simulink model "UKF_10hz"  (Simulink 8.3)
settings: Solver=FixedStepDiscrete  StartTime=0.0  StopTime=run_time  FixedStep=.01  RelTol=1e-3
values from neighbouring files (symbols this model uses):
  B_bias = [0 0 0]    [Initialize_UKF_Function.m]
  B_Init_Inertial = wrldmagm(Alt, Lat, Long, 2013)*1E-9    [Initialize_UKF_Function.m]
  I_c = [3.4 3.4 1.9]    [Initialize_UKF_Function.m]    (also in UKF_quaternion_withBias.m)
  NED_Init = dcmecef2ned(Lat, Long)*ECEF_Init    [Initialize_UKF_Function.m]
  q_i_s0 = init_attitude    [Initialize_UKF_Function.m]
  q_s_c = [1 0 0 0]    [Initialize_UKF_Function.m]    (also in Satellite2Controller_Conversion.m = dcm2quat(R); UKF_quaternion_withBias.m = [1; 0; 0; 0])
  Time_Start = 0    [Initialize_UKF_Function.m]
  Torque_s = [0 0 0]    [Initialize_UKF_Function.m]
  Ts = .1    (= 0.1)    [Initialize_UKF_Function.m]
  w_bias = 0*[0.5 0.2 0.15]    [Initialize_UKF_Function.m]    (also in UKF_quaternion_withBias.m = zeros(3,1))
  w_init_s = [rand_w_x rand_w_y rand_w_z]    [Initialize_UKF_Function.m]
undefined symbols (not defined in the file or in its folder): aeroassertmsg, c, cd, dyear, Earth, epoch, fm, fn, k, maxdef, Newton, Raphson, sgp4, snorm, WGS84
libraries: commnoisgen2 x6, aerolibtransform2 x4, aerolibconvert2 x4, simulink x3, dspmtrx3 x1, aerolibgravitysys x1, aerolibutil x1
(part 2 of 3)

== system UKF_10hz/Orbital Enviroment/Orbital Model/Subsystem/World Magnetic Model 2010/geomag/Rotate magnetic vector components  to geodetic from spherical and  compute declination, inclination  and total intensity/Compute declination, inclination,  and total intensity ==
  by : Inport
  bx : Inport  Port=2
  bz : Inport  Port=3
  Angle Conversion1 : aerolibconvert2/Angle Conversion  IU=rad  OU=deg
  Angle Conversion2 : aerolibconvert2/Angle Conversion  IU=rad  OU=deg
  Product : Product  SaturateOnIntegerOverflow=on  OutDataTypeStr=Inherit: Same as first input
  Product1 : Product  SaturateOnIntegerOverflow=on  OutDataTypeStr=Inherit: Same as first input
  Product2 : Product  SaturateOnIntegerOverflow=on  OutDataTypeStr=Inherit: Same as first input
  Sum : Sum  Inputs=|++  SaturateOnIntegerOverflow=on
  Sum1 : Sum  Inputs=++|  SaturateOnIntegerOverflow=on
  Trigonometric Function : Trigonometry  Operator=atan2
  Trigonometric Function1 : Trigonometry  Operator=atan2
  sqrt : Sqrt  AlgorithmType=Newton-Raphson  SaturateOnIntegerOverflow=on
  sqrt1 : Sqrt  AlgorithmType=Newton-Raphson  SaturateOnIntegerOverflow=on
  dec : Outport
  dip : Outport  Port=2
  ti : Outport  Port=3
  wires:
  sqrt/1 -> ti/1
  by/1 -> Product/1, Product/2, Trigonometric Function1/1
  bx/1 -> Product1/1, Product1/2, Trigonometric Function1/2
  bz/1 -> Product2/1, Product2/2, Trigonometric Function/1
  Product/1 -> Sum/1
  Product1/1 -> Sum/2
  Sum/1 -> Sum1/2, sqrt1/1
  Product2/1 -> Sum1/1
  Sum1/1 -> sqrt/1
  sqrt1/1 -> Trigonometric Function/2
  Trigonometric Function/1 -> Angle Conversion2/1
  Angle Conversion2/1 -> dip/1
  Trigonometric Function1/1 -> Angle Conversion1/1
  Angle Conversion1/1 -> dec/1

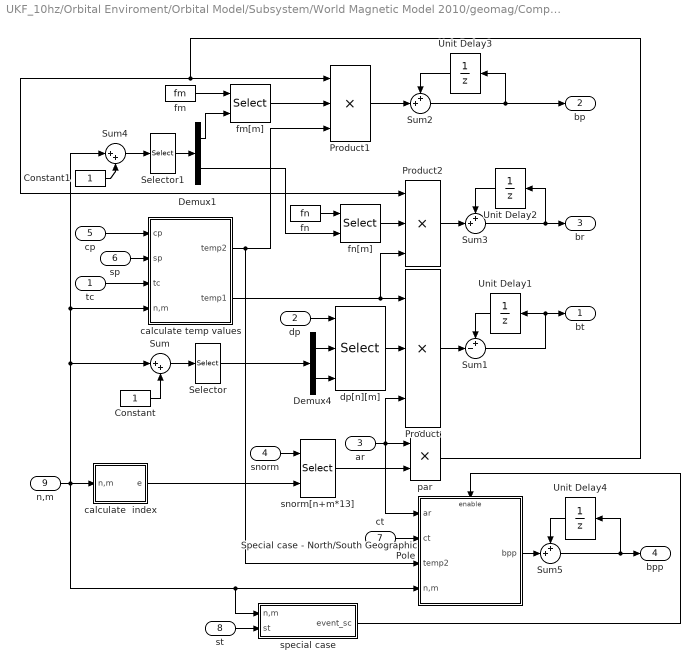
== system UKF_10hz/Orbital Enviroment/Orbital Model/Subsystem/World Magnetic Model 2010/geomag/Compute magnetic vector in spherical coordinates/For Iterator Subsystem/Accumulate terms of the  spherical harmonic expansion ==
  tc : Inport
  dp : Inport  Port=2
  ar : Inport  Port=3
  snorm : Inport  Port=4
  cp : Inport  Port=5
  sp : Inport  Port=6
  ct : Inport  Port=7
  st : Inport  Port=8
  n,m : Inport  Port=9
  Constant : Constant  OutDataTypeStr=Inherit: Inherit via back propagation
  Constant1 : Constant  OutDataTypeStr=Inherit: Inherit via back propagation
  Demux1 : Demux  Outputs=2
  Demux4 : Demux  Outputs=2
  Product : Product  Inputs=3  SaturateOnIntegerOverflow=on  OutDataTypeStr=Inherit: Same as first input
  Product1 : Product  Inputs=3  SaturateOnIntegerOverflow=on  OutDataTypeStr=Inherit: Same as first input
  Product2 : Product  Inputs=3  SaturateOnIntegerOverflow=on  OutDataTypeStr=Inherit: Same as first input
  Selector : Selector  InputPortWidth=2  Indices=[2 1]
  Selector1 : Selector  InputPortWidth=2  Indices=[2 1]
  Special case - North/South Geographic Pole : Subsystem  TreatAsAtomicUnit=on
  Sum : Sum  Inputs=|++  SaturateOnIntegerOverflow=on
  Sum1 : Sum  Inputs=+-|  SaturateOnIntegerOverflow=on
  Sum2 : Sum  Inputs=++|  SaturateOnIntegerOverflow=on
  Sum3 : Sum  Inputs=++|  SaturateOnIntegerOverflow=on
  Sum4 : Sum  Inputs=|++  SaturateOnIntegerOverflow=on
  Sum5 : Sum  Inputs=++|  SaturateOnIntegerOverflow=on
  Unit Delay{1..4} (4 alike) : UnitDelay  SampleTime=-1
  calculate  index : Subsystem
  calculate temp values : Subsystem
  dp[n][m] : Selector  NumberOfDimensions=2  InputPortWidth=maxdef+1  IndexOptions=Index vector (port),Index vector (port)  Indices=1,1
  fm : Constant  Value=fm  OutDataTypeStr=Inherit: Inherit via back propagation
  fm[m] : Selector  InputPortWidth=maxdef+1  IndexOptions=Index vector (port)  Indices=[1 3]
  fn : Constant  Value=fn  OutDataTypeStr=Inherit: Inherit via back propagation
  fn[m] : Selector  InputPortWidth=maxdef+1  IndexOptions=Index vector (port)  Indices=[1 3]
  par : Product  SaturateOnIntegerOverflow=on  OutDataTypeStr=Inherit: Same as first input
  snorm[n+m*13] : Selector  InputPortWidth=(maxdef+1)*(maxdef+1)  IndexOptions=Index vector (port)  Indices=[1 3]
  special case : Subsystem
  bt : Outport
  bp : Outport  Port=2
  br : Outport  Port=3
  bpp : Outport  Port=4
  wires:
  Special case - North/South Geographic Pole/1(bpp) -> Sum5/2
  Sum5/1 -> bpp/1, Unit Delay4/1
  Unit Delay4/1 -> Sum5/1
  snorm[n+m*13]/1 -> par/2
  ar/1 -> Product/3, par/1, Special case - North/South Geographic Pole/1(ar)
  calculate  index/1(e) -> snorm[n+m*13]/2
  calculate temp values/2(temp1) -> Product2/3, Product/1
  dp[n][m]/1 -> Product/2
  Product/1 -> Sum1/2
  Sum1/1 -> bt/1, Unit Delay1/1
  Unit Delay1/1 -> Sum1/1
  calculate temp values/1(temp2) -> Product1/3, Special case - North/South Geographic Pole/3(temp2)
  par/1 -> Product2/1, Product1/1
  fn/1 -> fn[m]/1
  fm/1 -> fm[m]/1
  Product1/1 -> Sum2/2
  Sum2/1 -> bp/1, Unit Delay3/1
  Unit Delay3/1 -> Sum2/1
  dp/1 -> dp[n][m]/1
  snorm/1 -> snorm[n+m*13]/1
  n,m/1 -> calculate  index/1(n,m), Sum/1, calculate temp values/4(n,m), Sum4/1, Special case - North/South Geographic Pole/4(n,m), special case/1(n,m)
  cp/1 -> calculate temp values/1(cp)
  sp/1 -> calculate temp values/2(sp)
  fn[m]/1 -> Product2/2
  fm[m]/1 -> Product1/2
  Product2/1 -> Sum3/2
  Sum3/1 -> br/1, Unit Delay2/1
  Unit Delay2/1 -> Sum3/1
  tc/1 -> calculate temp values/3(tc)
  Sum/1 -> Selector/1
  Constant/1 -> Sum/2
  Selector/1 -> Demux4/1
  Demux4/1 -> dp[n][m]/2
  Demux4/2 -> dp[n][m]/3
  Constant1/1 -> Sum4/2
  Sum4/1 -> Selector1/1
  Selector1/1 -> Demux1/1
  Demux1/1 -> fm[m]/2
  Demux1/2 -> fn[m]/2
  ct/1 -> Special case - North/South Geographic Pole/2(ct)
  st/1 -> special case/2(st)
  special case/1(event_sc) -> Special case - North/South Geographic Pole/Enable

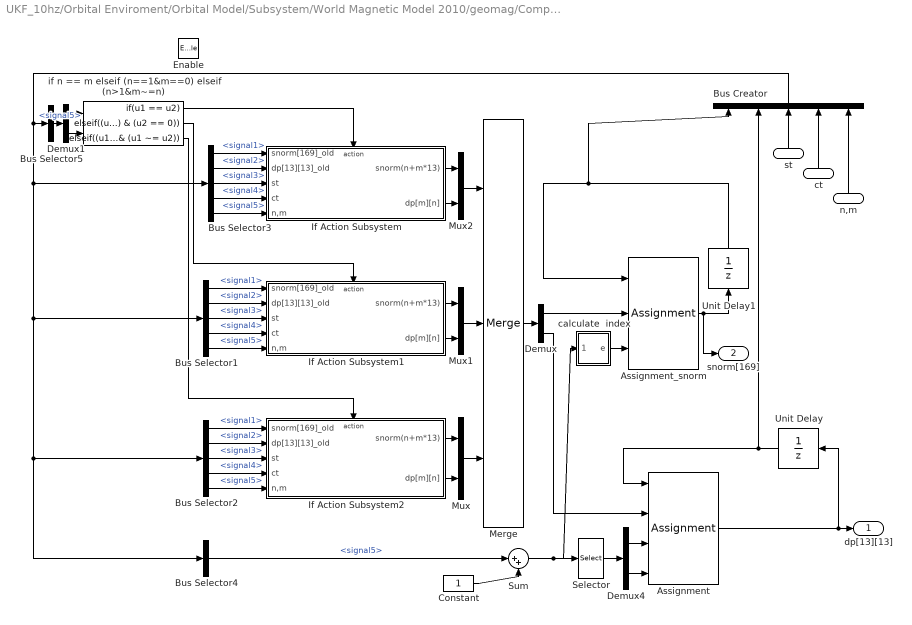
== system UKF_10hz/Orbital Enviroment/Orbital Model/Subsystem/World Magnetic Model 2010/geomag/Compute magnetic vector in spherical coordinates/For Iterator Subsystem/Compute unnormalized associated  legendre polynomials and  derivatives via recursion relations ==
  n,m : Inport
  st : Inport  Port=2
  ct : Inport  Port=3
  Enable : EnablePort  PropagateVarSize=During execution
  Assignment : Assignment  NumberOfDimensions=2  DiagnosticForDimensions=Error  IndexOptions=Index vector (port),Index vector (port)  Indices=1,1  OutputSizes=1,1
  Assignment_snorm : Assignment  DiagnosticForDimensions=Error  IndexOptions=Index vector (port)  OutputSizes=[1 1]
  Bus Creator : BusCreator  Inputs=5
  Bus Selector1 : BusSelector  OutputSignals=signal1,signal2,signal3,signal4,signal5
  Bus Selector2 : BusSelector  OutputSignals=signal1,signal2,signal3,signal4,signal5
  Bus Selector3 : BusSelector  OutputSignals=signal1,signal2,signal3,signal4,signal5
  Bus Selector4 : BusSelector  OutputSignals=signal5
  Bus Selector5 : BusSelector  OutputSignals=signal5
  Constant : Constant  OutDataTypeStr=Inherit: Inherit via back propagation
  Demux : Demux  Outputs=2
  Demux1 : Demux  Outputs=2
  Demux4 : Demux  Outputs=2
  If Action Subsystem : Subsystem  TreatAsAtomicUnit=on
  If Action Subsystem1 : Subsystem  TreatAsAtomicUnit=on
  If Action Subsystem2 : Subsystem  TreatAsAtomicUnit=on
  Merge : Merge  Inputs=3
  Mux : Mux  Inputs=2
  Mux1 : Mux  Inputs=2
  Mux2 : Mux  Inputs=2
  Selector : Selector  InputPortWidth=2  Indices=[2 1]
  Sum : Sum  Inputs=|++  SaturateOnIntegerOverflow=on
  Unit Delay : UnitDelay  InitialCondition=zeros(maxdef+1,maxdef+1)  SampleTime=-1
  Unit Delay1 : UnitDelay  InitialCondition=snorm  SampleTime=-1
  calculate  index : Subsystem
  if n == m elseif (n==1&m==0) elseif (n>1&m~=n) : If  NumInputs=2  IfExpression=u1 == u2  ElseIfExpressions=(u1 == 1) & (u2 == 0),(u1 >1) & (u1 ~= u2)  ShowElse=off
  dp[13][13] : Outport
  snorm[169] : Outport  Port=2
  wires:
  Constant/1 -> Sum/2
  if n == m elseif (n==1&m==0) elseif (n>1&m~=n)/1 -> If Action Subsystem/Action
  Assignment/1 -> dp[13][13]/1, Unit Delay/1
  if n == m elseif (n==1&m==0) elseif (n>1&m~=n)/2 -> If Action Subsystem1/Action
  if n == m elseif (n==1&m==0) elseif (n>1&m~=n)/3 -> If Action Subsystem2/Action
  Assignment_snorm/1 -> Unit Delay1/1, snorm[169]/1
  calculate  index/1(e) -> Assignment_snorm/3
  If Action Subsystem2/1(snorm(n+m*13)) -> Mux/1
  If Action Subsystem2/2(dp[m][n]) -> Mux/2
  If Action Subsystem1/1(snorm(n+m*13)) -> Mux1/1
  If Action Subsystem1/2(dp[m][n]) -> Mux1/2
  If Action Subsystem/1(snorm(n+m*13)) -> Mux2/1
  If Action Subsystem/2(dp[m][n]) -> Mux2/2
  Mux2/1 -> Merge/1
  Mux1/1 -> Merge/2
  Mux/1 -> Merge/3
  Merge/1 -> Demux/1
  Demux/2 -> Assignment/2
  Demux/1 -> Assignment_snorm/2
  Bus Selector2/1 -> If Action Subsystem2/1(snorm[169]_old)  "<signal1>"
  Bus Selector2/2 -> If Action Subsystem2/2(dp[13][13]_old)  "<signal2>"
  Bus Selector2/3 -> If Action Subsystem2/3(st)  "<signal3>"
  Bus Selector2/4 -> If Action Subsystem2/4(ct)  "<signal4>"
  Bus Selector1/1 -> If Action Subsystem1/1(snorm[169]_old)  "<signal1>"
  Bus Selector1/2 -> If Action Subsystem1/2(dp[13][13]_old)  "<signal2>"
  Bus Selector1/3 -> If Action Subsystem1/3(st)  "<signal3>"
  Bus Selector1/4 -> If Action Subsystem1/4(ct)  "<signal4>"
  Bus Selector3/1 -> If Action Subsystem/1(snorm[169]_old)  "<signal1>"
  Bus Selector3/2 -> If Action Subsystem/2(dp[13][13]_old)  "<signal2>"
  Bus Selector3/3 -> If Action Subsystem/3(st)  "<signal3>"
  Bus Selector3/4 -> If Action Subsystem/4(ct)  "<signal4>"
  st/1 -> Bus Creator/3
  ct/1 -> Bus Creator/4
  Bus Creator/1 -> Bus Selector1/1, Bus Selector2/1, Bus Selector4/1, Bus Selector3/1, Bus Selector5/1
  Sum/1 -> calculate  index/1(n,m), Selector/1
  Demux4/1 -> Assignment/3
  Demux4/2 -> Assignment/4
  Selector/1 -> Demux4/1
  n,m/1 -> Bus Creator/5
  Bus Selector1/5 -> If Action Subsystem1/5(n,m)  "<signal5>"
  Bus Selector2/5 -> If Action Subsystem2/5(n,m)  "<signal5>"
  Bus Selector3/5 -> If Action Subsystem/5(n,m)  "<signal5>"
  Bus Selector4/1 -> Sum/1  "<signal5>"
  Unit Delay/1 -> Assignment/1, Bus Creator/2
  Unit Delay1/1 -> Bus Creator/1, Assignment_snorm/1
  Demux1/1 -> if n == m elseif (n==1&m==0) elseif (n>1&m~=n)/1
  Demux1/2 -> if n == m elseif (n==1&m==0) elseif (n>1&m~=n)/2
  Bus Selector5/1 -> Demux1/1  "<signal5>"

== system UKF_10hz/Orbital Enviroment/Orbital Model/Subsystem/World Magnetic Model 2010/geomag/Compute magnetic vector in spherical coordinates/For Iterator Subsystem/Time adjust the gauss coefficients ==
  n : Inport
  m : Inport  Port=2
  dt : Inport  Port=3
  Enable : EnablePort  PropagateVarSize=During execution
  Assignment : Assignment  NumberOfDimensions=2  DiagnosticForDimensions=Error  IndexOptions=Index vector (port),Index vector (port)  Indices=1,1  OutputSizes=1,1
  Bus Creator : BusCreator  Inputs=5
  Bus Selector1 : BusSelector  OutputSignals=signal1,signal2,signal3,signal4,signal5
  If Action Subsystem : Subsystem  TreatAsAtomicUnit=on
  Sum2 : Sum  Inputs=|++  OutDataTypeStr=Inherit: Inherit via back propagation  SaturateOnIntegerOverflow=on
  Unit Delay : UnitDelay  InitialCondition=zeros(maxdef+1,maxdef+1)  SampleTime=-1
  c[maxdef][maxdef] : Constant  Value=c  OutDataTypeStr=Inherit: Inherit via back propagation
  cd[maxdef][maxdef] : Constant  Value=cd  OutDataTypeStr=Inherit: Inherit via back propagation
  if (m~=0) : Subsystem
  tc[13][13] : Outport
  wires:
  m/1 -> Bus Creator/1
  Bus Selector1/1 -> If Action Subsystem/1(m)  "<signal1>"
  Bus Selector1/2 -> If Action Subsystem/2(n)  "<signal2>"
  Bus Selector1/3 -> If Action Subsystem/3(dt)  "<signal3>"
  Bus Selector1/5 -> If Action Subsystem/5(cd)  "<signal5>"
  n/1 -> Bus Creator/2
  dt/1 -> Bus Creator/3
  c[maxdef][maxdef]/1 -> Bus Creator/4
  cd[maxdef][maxdef]/1 -> Bus Creator/5
  Assignment/1 -> Unit Delay/1, Sum2/1
  If Action Subsystem/1(tc) -> Assignment/2
  If Action Subsystem/2(row) -> Assignment/3
  If Action Subsystem/3(col) -> Assignment/4
  Bus Creator/1 -> if (m~=0)/1(bus), Bus Selector1/1
  Bus Selector1/4 -> If Action Subsystem/4(c)  "<signal4>"
  if (m~=0)/1(tc[13][13]) -> Sum2/2
  Unit Delay/1 -> Assignment/1
  Sum2/1 -> tc[13][13]/1

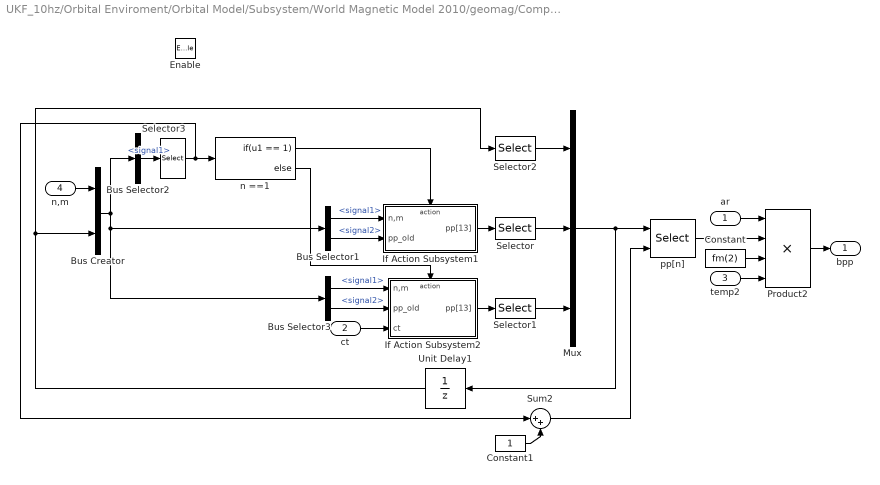
== system UKF_10hz/Orbital Enviroment/Orbital Model/Subsystem/World Magnetic Model 2010/geomag/Compute magnetic vector in spherical coordinates/For Iterator Subsystem/Accumulate terms of the  spherical harmonic expansion/Special case - North/South Geographic Pole ==
  ar : Inport
  ct : Inport  Port=2
  temp2 : Inport  Port=3
  n,m : Inport  Port=4
  Enable : EnablePort  PropagateVarSize=During execution
  Bus Creator : BusCreator  Inputs=2
  Bus Selector1 : BusSelector  OutputSignals=signal1,signal2
  Bus Selector2 : BusSelector  OutputSignals=signal1
  Bus Selector3 : BusSelector  OutputSignals=signal1,signal2
  Constant : Constant  Value=fm(2)  OutDataTypeStr=Inherit: Inherit via back propagation
  Constant1 : Constant
  If Action Subsystem1 : Subsystem
  If Action Subsystem2 : Subsystem
  Mux : Mux  Inputs=3
  Product2 : Product  Inputs=4  SaturateOnIntegerOverflow=on  OutDataTypeStr=Inherit: Same as first input
  Selector : Selector  InputPortWidth=maxdef+1  Indices=[2]
  Selector1 : Selector  InputPortWidth=maxdef+1  Indices=3:maxdef+1
  Selector2 : Selector  InputPortWidth=maxdef+1  Indices=[1]
  Selector3 : Selector  InputPortWidth=2
  Sum2 : Sum  Inputs=|++  SaturateOnIntegerOverflow=on
  Unit Delay1 : UnitDelay  InitialCondition=ones(1,maxdef+1)  SampleTime=-1
  n ==1 : If  IfExpression=u1 == 1
  pp[n] : Selector  InputPortWidth=maxdef+1  IndexOptions=Index vector (port)  Indices=[1 3]
  bpp : Outport  OutputWhenDisabled=reset  InitialOutput=0
  wires:
  Selector2/1 -> Mux/1
  Selector1/1 -> Mux/3
  Selector/1 -> Mux/2
  Mux/1 -> pp[n]/1, Unit Delay1/1
  n,m/1 -> Bus Creator/1
  ar/1 -> Product2/1
  Bus Creator/1 -> Bus Selector2/1, Bus Selector1/1, Bus Selector3/1
  Bus Selector2/1 -> Selector3/1  "<signal1>"
  If Action Subsystem1/1(pp[13]) -> Selector/1
  If Action Subsystem2/1(pp[13]) -> Selector1/1
  n ==1/1 -> If Action Subsystem1/Action
  n ==1/2 -> If Action Subsystem2/Action
  ct/1 -> If Action Subsystem2/3(ct)
  Unit Delay1/1 -> Selector2/1, Bus Creator/2
  Bus Selector1/1 -> If Action Subsystem1/1(n,m)  "<signal1>"
  Bus Selector1/2 -> If Action Subsystem1/2(pp_old)  "<signal2>"
  Bus Selector3/1 -> If Action Subsystem2/1(n,m)  "<signal1>"
  Bus Selector3/2 -> If Action Subsystem2/2(pp_old)  "<signal2>"
  Constant/1 -> Product2/3
  temp2/1 -> Product2/4
  Product2/1 -> bpp/1
  pp[n]/1 -> Product2/2
  Sum2/1 -> pp[n]/2
  Constant1/1 -> Sum2/2
  Selector3/1 -> n ==1/1, Sum2/1

== system UKF_10hz/Orbital Enviroment/Orbital Model/Subsystem/World Magnetic Model 2010/geomag/Compute magnetic vector in spherical coordinates/For Iterator Subsystem/Accumulate terms of the  spherical harmonic expansion/calculate  index ==
  n,m : Inport
  Constant : Constant  OutDataTypeStr=Inherit: Inherit via back propagation
  Demux8 : Demux  Outputs=2
  Gain : Gain  Gain=maxdef+1  SaturateOnIntegerOverflow=on  OutDataTypeStr=Inherit: Same as input  ParamDataTypeStr=Inherit: Same as input
  Sum1 : Sum  Inputs=+++  SaturateOnIntegerOverflow=on
  e : Outport
  wires:
  Gain/1 -> Sum1/3
  Demux8/1 -> Sum1/2
  Demux8/2 -> Gain/1
  n,m/1 -> Demux8/1
  Sum1/1 -> e/1
  Constant/1 -> Sum1/1

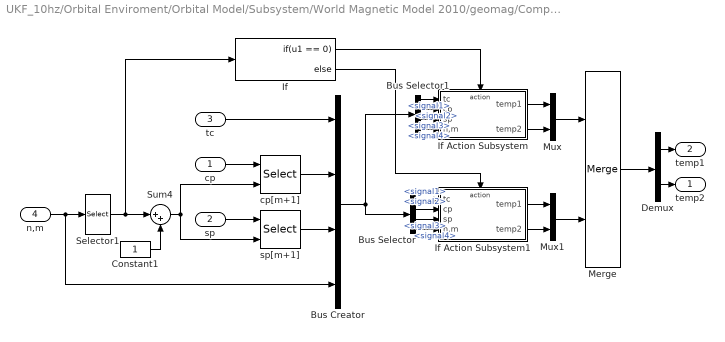
== system UKF_10hz/Orbital Enviroment/Orbital Model/Subsystem/World Magnetic Model 2010/geomag/Compute magnetic vector in spherical coordinates/For Iterator Subsystem/Accumulate terms of the  spherical harmonic expansion/calculate temp values ==
  cp : Inport
  sp : Inport  Port=2
  tc : Inport  Port=3
  n,m : Inport  Port=4
  Bus Creator : BusCreator
  Bus Selector : BusSelector  OutputSignals=signal1,signal2,signal3,signal4
  Bus Selector1 : BusSelector  OutputSignals=signal1,signal2,signal3,signal4
  Constant1 : Constant
  Demux : Demux  Outputs=2
  If : If  IfExpression=u1 == 0
  If Action Subsystem : Subsystem  TreatAsAtomicUnit=on
  If Action Subsystem1 : Subsystem  TreatAsAtomicUnit=on
  Merge : Merge
  Mux : Mux  Inputs=2
  Mux1 : Mux  Inputs=2
  Selector1 : Selector  InputPortWidth=2  Indices=2
  Sum4 : Sum  Inputs=|++  SaturateOnIntegerOverflow=on
  cp[m+1] : Selector  InputPortWidth=maxdef+1  IndexOptions=Index vector (port)  Indices=[1 3]
  sp[m+1] : Selector  InputPortWidth=maxdef+1  IndexOptions=Index vector (port)  Indices=[1 3]
  temp2 : Outport
  temp1 : Outport  Port=2
  wires:
  sp/1 -> sp[m+1]/1
  cp/1 -> cp[m+1]/1
  Selector1/1 -> Sum4/1, If/1
  Constant1/1 -> Sum4/2
  Sum4/1 -> sp[m+1]/2, cp[m+1]/2
  n,m/1 -> Selector1/1, Bus Creator/4
  If/1 -> If Action Subsystem/Action
  Bus Selector1/1 -> If Action Subsystem/1(tc)  "<signal1>"
  Bus Selector1/2 -> If Action Subsystem/2(cp)  "<signal2>"
  Bus Selector1/3 -> If Action Subsystem/3(sp)  "<signal3>"
  If/2 -> If Action Subsystem1/Action
  Bus Selector/1 -> If Action Subsystem1/1(tc)  "<signal1>"
  Bus Selector/2 -> If Action Subsystem1/2(cp)  "<signal2>"
  Bus Selector/3 -> If Action Subsystem1/3(sp)  "<signal3>"
  Demux/1 -> temp1/1
  Demux/2 -> temp2/1
  Merge/1 -> Demux/1
  If Action Subsystem/1(temp1) -> Mux/1
  If Action Subsystem/2(temp2) -> Mux/2
  If Action Subsystem1/1(temp1) -> Mux1/1
  If Action Subsystem1/2(temp2) -> Mux1/2
  Mux/1 -> Merge/1
  Mux1/1 -> Merge/2
  tc/1 -> Bus Creator/1
  cp[m+1]/1 -> Bus Creator/2
  sp[m+1]/1 -> Bus Creator/3
  Bus Creator/1 -> Bus Selector/1, Bus Selector1/1
  Bus Selector1/4 -> If Action Subsystem/4(n,m)  "<signal4>"
  Bus Selector/4 -> If Action Subsystem1/4(n,m)  "<signal4>"

== system UKF_10hz/Orbital Enviroment/Orbital Model/Subsystem/World Magnetic Model 2010/geomag/Compute magnetic vector in spherical coordinates/For Iterator Subsystem/Accumulate terms of the  spherical harmonic expansion/special case ==
  n,m : Inport
  st : Inport  Port=2
  Constant : Constant  OutDataTypeStr=Inherit: Inherit via back propagation
  Constant1 : Constant  Value=0
  Logical Operator : Logic  AllPortsSameDT=off
  Relational Operator : RelationalOperator  Operator===
  Relational Operator1 : RelationalOperator  Operator===
  Selector2 : Selector  InputPortWidth=2  Indices=2
  event_sc : Outport
  wires:
  n,m/1 -> Selector2/1
  Selector2/1 -> Relational Operator/2
  Logical Operator/1 -> event_sc/1
  st/1 -> Relational Operator1/1
  Constant/1 -> Relational Operator/1
  Constant1/1 -> Relational Operator1/2
  Relational Operator1/1 -> Logical Operator/1
  Relational Operator/1 -> Logical Operator/2

== system UKF_10hz/Orbital Enviroment/Orbital Model/Subsystem/World Magnetic Model 2010/geomag/Compute magnetic vector in spherical coordinates/For Iterator Subsystem/Compute unnormalized associated  legendre polynomials and  derivatives via recursion relations/If Action Subsystem ==
  snorm[169]_old : Inport
  dp[13][13]_old : Inport  Port=2
  st : Inport  Port=3
  ct : Inport  Port=4
  n,m : Inport  Port=5
  Action Port : ActionPort  PropagateVarSize=During execution  ActionType=then
  Product : Product  SaturateOnIntegerOverflow=on  OutDataTypeStr=Inherit: Same as first input
  Product1 : Product  SaturateOnIntegerOverflow=on  OutDataTypeStr=Inherit: Same as first input
  Product2 : Product  SaturateOnIntegerOverflow=on  OutDataTypeStr=Inherit: Same as first input
  Reshape : Reshape
  Selector : Selector  InputPortWidth=(maxdef+1)*(maxdef+1)  IndexOptions=Index vector (port)  Indices=[1 3]
  Selector1 : Selector  NumberOfDimensions=2  InputPortWidth=(maxdef+1)*(maxdef+1)  IndexOptions=Index vector (port),Index vector (port)  Indices=1,1
  Sum : Sum  Inputs=|++  SaturateOnIntegerOverflow=on
  calculate  index : Subsystem
  calculate  row and column : Subsystem
  snorm(n+m*13) : Outport
  dp[m][n] : Outport  Port=2
  wires:
  n,m/1 -> calculate  index/1(n,m), calculate  row and column/1(n,m)
  calculate  index/1(e) -> Selector/2
  snorm[169]_old/1 -> Selector/1
  dp[13][13]_old/1 -> Selector1/1
  calculate  row and column/1(m) -> Selector1/2
  Selector1/1 -> Reshape/1
  st/1 -> Product/1, Product1/1
  Sum/1 -> dp[m][n]/1
  Product/1 -> Sum/2
  Selector/1 -> Product1/2, Product2/2
  Product1/1 -> snorm(n+m*13)/1
  ct/1 -> Product2/1
  Product2/1 -> Sum/1
  calculate  row and column/2(n) -> Selector1/3
  Reshape/1 -> Product/2

== system UKF_10hz/Orbital Enviroment/Orbital Model/Subsystem/World Magnetic Model 2010/geomag/Compute magnetic vector in spherical coordinates/For Iterator Subsystem/Compute unnormalized associated  legendre polynomials and  derivatives via recursion relations/If Action Subsystem1 ==
  snorm[169]_old : Inport
  dp[13][13]_old : Inport  Port=2
  st : Inport  Port=3
  ct : Inport  Port=4
  n,m : Inport  Port=5
  Action Port : ActionPort  PropagateVarSize=During execution  ActionType=elseif
  Product : Product  SaturateOnIntegerOverflow=on  OutDataTypeStr=Inherit: Same as first input
  Product2 : Product  SaturateOnIntegerOverflow=on  OutDataTypeStr=Inherit: Same as first input
  Product3 : Product  SaturateOnIntegerOverflow=on  OutDataTypeStr=Inherit: Same as first input
  Reshape : Reshape
  Selector : Selector  InputPortWidth=(maxdef+1)*(maxdef+1)  IndexOptions=Index vector (port)  Indices=[1 3]
  Selector1 : Selector  NumberOfDimensions=2  InputPortWidth=(maxdef+1)*(maxdef+1)  IndexOptions=Index vector (port),Index vector (port)  Indices=1,1
  Sum : Sum  Inputs=|-+  SaturateOnIntegerOverflow=on
  calculate  index : Subsystem
  calculate  row and column : Subsystem
  snorm(n+m*13) : Outport
  dp[m][n] : Outport  Port=2
  wires:
  n,m/1 -> calculate  index/1(n,m), calculate  row and column/1(n,m)
  calculate  index/1(e) -> Selector/2
  snorm[169]_old/1 -> Selector/1
  dp[13][13]_old/1 -> Selector1/1
  Selector1/1 -> Reshape/1
  ct/1 -> Product/1, Product3/1
  Product/1 -> Sum/2
  Selector/1 -> Product2/2, Product3/2
  Product3/1 -> snorm(n+m*13)/1
  st/1 -> Product2/1
  Product2/1 -> Sum/1
  Sum/1 -> dp[m][n]/1
  calculate  row and column/1(m+1) -> Selector1/2
  calculate  row and column/2(n) -> Selector1/3
  Reshape/1 -> Product/2

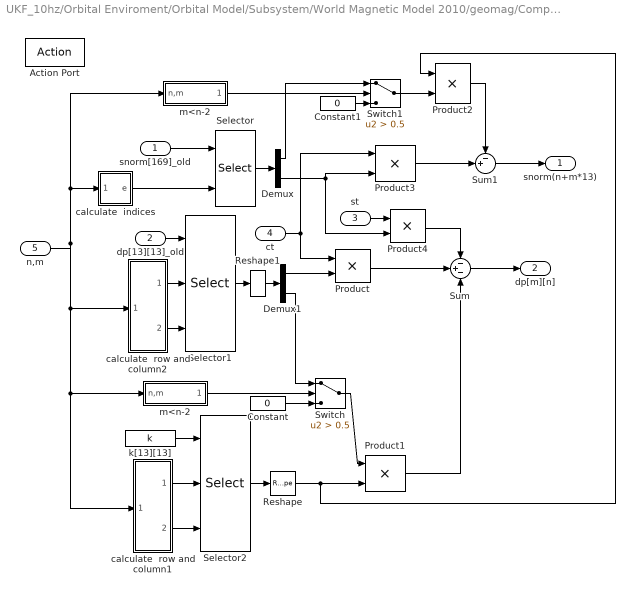
== system UKF_10hz/Orbital Enviroment/Orbital Model/Subsystem/World Magnetic Model 2010/geomag/Compute magnetic vector in spherical coordinates/For Iterator Subsystem/Compute unnormalized associated  legendre polynomials and  derivatives via recursion relations/If Action Subsystem2 ==
  snorm[169]_old : Inport
  dp[13][13]_old : Inport  Port=2
  st : Inport  Port=3
  ct : Inport  Port=4
  n,m : Inport  Port=5
  Action Port : ActionPort  PropagateVarSize=During execution  ActionType=elseif
  Constant : Constant  Value=0  OutDataTypeStr=Inherit: Inherit via back propagation
  Constant1 : Constant  Value=0  OutDataTypeStr=Inherit: Inherit via back propagation
  Demux : Demux  Outputs=2
  Demux1 : Demux  Outputs=2
  Product{,1..4} (5 alike) : Product  SaturateOnIntegerOverflow=on  OutDataTypeStr=Inherit: Same as first input
  Reshape : Reshape
  Reshape1 : Reshape
  Selector : Selector  InputPortWidth=(maxdef+1)*(maxdef+1)  IndexOptions=Index vector (port)  Indices=[1 3]
  Selector1 : Selector  NumberOfDimensions=2  InputPortWidth=(maxdef+1)*(maxdef+1)  IndexOptions=Index vector (port),Index vector (port)  Indices=1,1
  Selector2 : Selector  NumberOfDimensions=2  InputPortWidth=(maxdef+1)*(maxdef+1)  IndexOptions=Index vector (port),Index vector (port)  Indices=1,1
  Sum : Sum  Inputs=-+-  SaturateOnIntegerOverflow=on
  Sum1 : Sum  Inputs=-+|  SaturateOnIntegerOverflow=on
  Switch : Switch  Criteria=u2 > Threshold  Threshold=0.5  SaturateOnIntegerOverflow=on
  Switch1 : Switch  Criteria=u2 > Threshold  Threshold=0.5  SaturateOnIntegerOverflow=on
  calculate  indices : Subsystem
  calculate  row and column1 : Subsystem
  calculate  row and column2 : Subsystem
  k[13][13] : Constant  Value=k  OutDataTypeStr=Inherit: Inherit via back propagation
  m<n-2 : Subsystem
  "m<n-2 " : Subsystem
  snorm(n+m*13) : Outport
  dp[m][n] : Outport  Port=2
  wires:
  n,m/1 -> calculate  row and column1/1(n,m), m<n-2/1(n,m), calculate  row and column2/1(n,m), calculate  indices/1(n,m), "m<n-2 "/1(n,m)
  calculate  indices/1(e) -> Selector/2
  snorm[169]_old/1 -> Selector/1
  dp[13][13]_old/1 -> Selector1/1
  Selector1/1 -> Reshape1/1
  ct/1 -> Product/1, Product3/1
  Product/1 -> Sum/2
  Product3/1 -> Sum1/2
  st/1 -> Product4/1
  Product4/1 -> Sum/1
  calculate  row and column2/1(m+1) -> Selector1/2
  calculate  row and column2/2(n-1,n) -> Selector1/3
  k[13][13]/1 -> Selector2/1
  calculate  row and column1/1(m+1) -> Selector2/2
  calculate  row and column1/2(n+1) -> Selector2/3
  Selector/1 -> Demux/1
  Selector2/1 -> Reshape/1
  Demux1/1 -> Product/2
  Product1/1 -> Sum/3
  Demux1/2 -> Switch/1
  Switch/1 -> Product1/1
  Constant/1 -> Switch/3
  m<n-2/1(n-2>=m) -> Switch/2
  Sum/1 -> dp[m][n]/1
  Demux/2 -> Product3/2, Product4/2
  Demux/1 -> Switch1/1
  Constant1/1 -> Switch1/3
  Sum1/1 -> snorm(n+m*13)/1
  Reshape/1 -> Product1/2, Product2/1
  Reshape1/1 -> Demux1/1
  Product2/1 -> Sum1/1
  Switch1/1 -> Product2/2
  "m<n-2 "/1(n-2>=m) -> Switch1/2

== system UKF_10hz/Orbital Enviroment/Orbital Model/Subsystem/World Magnetic Model 2010/geomag/Compute magnetic vector in spherical coordinates/For Iterator Subsystem/Compute unnormalized associated  legendre polynomials and  derivatives via recursion relations/calculate  index ==
  n,m : Inport
  Constant : Constant  OutDataTypeStr=Inherit: Inherit via back propagation
  Demux8 : Demux  Outputs=2
  Gain : Gain  Gain=maxdef+1  SaturateOnIntegerOverflow=on  OutDataTypeStr=Inherit: Same as input  ParamDataTypeStr=Inherit: Same as input
  Sum1 : Sum  Inputs=|++  OutDataTypeStr=Inherit: Inherit via back propagation  SaturateOnIntegerOverflow=on
  Sum2 : Sum  Inputs=|+-  SaturateOnIntegerOverflow=on
  e : Outport
  wires:
  Gain/1 -> Sum1/2
  Demux8/1 -> Sum1/1
  n,m/1 -> Demux8/1
  Sum1/1 -> e/1
  Demux8/2 -> Sum2/1
  Sum2/1 -> Gain/1
  Constant/1 -> Sum2/2

== system UKF_10hz/Orbital Enviroment/Orbital Model/Subsystem/World Magnetic Model 2010/geomag/Compute magnetic vector in spherical coordinates/For Iterator Subsystem/Time adjust the gauss coefficients/If Action Subsystem ==
  m : Inport
  n : Inport  Port=2
  dt : Inport  Port=3
  c : Inport  Port=4
  cd : Inport  Port=5
  Constant : Constant  OutDataTypeStr=Inherit: Inherit via back propagation
  Constant1 : Constant  OutDataTypeStr=Inherit: Inherit via back propagation
  Product : Product  SaturateOnIntegerOverflow=on  OutDataTypeStr=Inherit: Same as first input
  Sum : Sum  Inputs=|++  OutDataTypeStr=Inherit: Inherit via back propagation  SaturateOnIntegerOverflow=on
  Sum1 : Sum  Inputs=|++  SaturateOnIntegerOverflow=on  InputSameDT=on
  Sum2 : Sum  Inputs=|++  SaturateOnIntegerOverflow=on  InputSameDT=on
  c[m][n] : Selector  NumberOfDimensions=2  InputPortWidth=3  IndexOptions=Index vector (port),Index vector (port)  Indices=1,1
  cd[m][n] : Selector  NumberOfDimensions=2  InputPortWidth=3  IndexOptions=Index vector (port),Index vector (port)  Indices=1,1
  tc : Outport
  row : Outport  Port=2
  col : Outport  Port=3
  wires:
  c/1 -> c[m][n]/1
  Sum1/1 -> c[m][n]/2, row/1, cd[m][n]/2
  Sum2/1 -> c[m][n]/3, col/1, cd[m][n]/3
  cd/1 -> cd[m][n]/1
  dt/1 -> Product/2
  cd[m][n]/1 -> Product/1
  c[m][n]/1 -> Sum/1
  Product/1 -> Sum/2
  Sum/1 -> tc/1
  Constant/1 -> Sum2/2
  n/1 -> Sum2/1
  Constant1/1 -> Sum1/2
  m/1 -> Sum1/1

== system UKF_10hz/Orbital Enviroment/Orbital Model/Subsystem/World Magnetic Model 2010/geomag/Compute magnetic vector in spherical coordinates/For Iterator Subsystem/Time adjust the gauss coefficients/if (m~=0) ==
  bus : Inport
  Bus Selector : BusSelector  OutputSignals=signal1,signal2,signal3,signal4,signal5
  Bus Selector1 : BusSelector  OutputSignals=signal2
  Bus Selector2 : BusSelector  OutputSignals=signal1
  If : If  IfExpression=u1 ~= 0
  If Action Subsystem1 : Subsystem
  If Action Subsystem2 : Subsystem
  Merge : Merge
  Unit Delay : UnitDelay  InitialCondition=zeros(maxdef+1,maxdef+1)  SampleTime=-1
  tc_old : Switch  Criteria=u2 > Threshold  Threshold=1  SaturateOnIntegerOverflow=on
  zeros(maxdef+1,maxdef+1) : Constant  Value=zeros(maxdef+1,maxdef+1)  OutDataTypeStr=Inherit: Inherit via back propagation
  tc[13][13] : Outport
  wires:
  Bus Selector/1 -> If Action Subsystem1/1(m)  "<signal1>"
  Bus Selector/2 -> If Action Subsystem1/2(n)  "<signal2>"
  Bus Selector/3 -> If Action Subsystem1/3(dt)  "<signal3>"
  Bus Selector/4 -> If Action Subsystem1/4(c)  "<signal4>"
  Bus Selector/5 -> If Action Subsystem1/5(cd)  "<signal5>"
  If/1 -> If Action Subsystem1/Action
  Bus Selector2/1 -> If/1  "<signal1>"
  bus/1 -> Bus Selector2/1, Bus Selector/1, Bus Selector1/1
  Merge/1 -> tc[13][13]/1, Unit Delay/1
  If Action Subsystem1/1(tc[13][13]) -> Merge/1
  If Action Subsystem2/1(tc[13][13]) -> Merge/2
  If/2 -> If Action Subsystem2/Action
  tc_old/1 -> If Action Subsystem2/1(tc_old), If Action Subsystem1/6(tc_old)
  Bus Selector1/1 -> tc_old/2  "<signal2>"
  zeros(maxdef+1,maxdef+1)/1 -> tc_old/3
  Unit Delay/1 -> tc_old/1

== system UKF_10hz/Orbital Enviroment/Orbital Model/Subsystem/World Magnetic Model 2010/geomag/Compute magnetic vector in spherical coordinates/For Iterator Subsystem/Accumulate terms of the  spherical harmonic expansion/Special case - North/South Geographic Pole/If Action Subsystem1 ==
  n,m : Inport
  pp_old : Inport  Port=2
  Action Port : ActionPort  PropagateVarSize=During execution  ActionType=then
  Assignment2 : Assignment  DiagnosticForDimensions=Error  IndexOptions=Index vector (port)  OutputSizes=[1 1]
  Constant : Constant
  Selector3 : Selector  InputPortWidth=2
  Sum2 : Sum  Inputs=|++  SaturateOnIntegerOverflow=on
  pp[n-1] : Selector  InputPortWidth=maxdef+1  IndexOptions=Index vector (port)  Indices=[1 3]
  pp[13] : Outport
  wires:
  Assignment2/1 -> pp[13]/1
  pp_old/1 -> Assignment2/1, pp[n-1]/1
  n,m/1 -> Selector3/1
  Constant/1 -> Sum2/2
  Sum2/1 -> Assignment2/3
  pp[n-1]/1 -> Assignment2/2
  Selector3/1 -> Sum2/1, pp[n-1]/2

== system UKF_10hz/Orbital Enviroment/Orbital Model/Subsystem/World Magnetic Model 2010/geomag/Compute magnetic vector in spherical coordinates/For Iterator Subsystem/Accumulate terms of the  spherical harmonic expansion/Special case - North/South Geographic Pole/If Action Subsystem2 ==
  n,m : Inport
  pp_old : Inport  Port=2
  ct : Inport  Port=3
  Action Port : ActionPort  PropagateVarSize=During execution  ActionType=else
  Assignment2 : Assignment  DiagnosticForDimensions=Error  IndexOptions=Index vector (port)  OutputSizes=[1 1]
  Constant : Constant  OutDataTypeStr=Inherit: Inherit via back propagation
  Demux8 : Demux  Outputs=2
  Product1 : Product  OutDataTypeStr=Inherit: Inherit via back propagation  SaturateOnIntegerOverflow=on  InputSameDT=on
  Product2 : Product  SaturateOnIntegerOverflow=on  OutDataTypeStr=Inherit: Same as first input
  Reshape : Reshape
  Selector1 : Selector  InputPortWidth=2
  Selector2 : Selector  NumberOfDimensions=2  InputPortWidth=(maxdef+1)*(maxdef+1)  IndexOptions=Index vector (port),Index vector (port)  Indices=1,1
  Sum1 : Sum  Inputs=|+-  SaturateOnIntegerOverflow=on  OutDataTypeStr=Inherit: Same as first input
  Sum2 : Sum  Inputs=|++  SaturateOnIntegerOverflow=on  InputSameDT=on
  calculate  indices : Subsystem
  calculate  row and column : Subsystem
  k[13][13] : Constant  Value=k  OutDataTypeStr=Inherit: Inherit via back propagation
  pp[n-2] pp[n-1] : Selector  InputPortWidth=maxdef+1  IndexOptions=Index vector (port)  Indices=[1 3]
  pp[13] : Outport
  wires:
  n,m/1 -> calculate  row and column/1(n,m), Selector1/1
  Constant/1 -> Sum2/2
  Sum2/1 -> Assignment2/3
  pp_old/1 -> pp[n-2] pp[n-1]/1, Assignment2/1
  Assignment2/1 -> pp[13]/1
  calculate  indices/1(e) -> pp[n-2] pp[n-1]/2
  pp[n-2] pp[n-1]/1 -> Demux8/1
  ct/1 -> Product2/1
  Demux8/2 -> Product2/2
  Product2/1 -> Sum1/1
  Sum1/1 -> Assignment2/2
  Demux8/1 -> Product1/2
  Product1/1 -> Sum1/2
  k[13][13]/1 -> Selector2/1
  calculate  row and column/1(m+1) -> Selector2/2
  calculate  row and column/2(n+1) -> Selector2/3
  Selector2/1 -> Reshape/1
  Reshape/1 -> Product1/1
  Selector1/1 -> Sum2/1, calculate  indices/1(n)

== system UKF_10hz/Orbital Enviroment/Orbital Model/Subsystem/World Magnetic Model 2010/geomag/Compute magnetic vector in spherical coordinates/For Iterator Subsystem/Accumulate terms of the  spherical harmonic expansion/calculate temp values/If Action Subsystem ==
  tc : Inport
  cp : Inport  Port=2
  sp : Inport  Port=3
  n,m : Inport  Port=4
  Action Port : ActionPort  PropagateVarSize=During execution  ActionType=then
  Constant : Constant
  Demux : Demux  Outputs=2
  Demux1 : Demux  Outputs=2
  Mux : Mux  Inputs=2
  Product : Product  SaturateOnIntegerOverflow=on  InputSameDT=on  OutDataTypeStr=Inherit: Same as first input
  Selector : Selector  NumberOfDimensions=2  InputPortWidth=3  IndexOptions=Index vector (port),Index vector (port)  Indices=1,1
  Selector1 : Selector  InputPortWidth=2  Indices=[2 1]
  Sum : Sum  Inputs=|++  SaturateOnIntegerOverflow=on
  temp1 : Outport
  temp2 : Outport  Port=2
  wires:
  cp/1 -> Mux/1
  sp/1 -> Mux/2
  tc/1 -> Selector/1
  Selector/1 -> Product/2
  Demux/1 -> Selector/2
  Demux/2 -> Selector/3
  Sum/1 -> Selector1/1
  n,m/1 -> Sum/1
  Constant/1 -> Sum/2
  Selector1/1 -> Demux/1
  Mux/1 -> Product/1
  Product/1 -> Demux1/1
  Demux1/1 -> temp1/1
  Demux1/2 -> temp2/1

== system UKF_10hz/Orbital Enviroment/Orbital Model/Subsystem/World Magnetic Model 2010/geomag/Compute magnetic vector in spherical coordinates/For Iterator Subsystem/Accumulate terms of the  spherical harmonic expansion/calculate temp values/If Action Subsystem1 ==
  tc : Inport
  cp : Inport  Port=2
  sp : Inport  Port=3
  n,m : Inport  Port=4
  Action Port : ActionPort  PropagateVarSize=During execution  ActionType=else
  Demux1 : Demux  Outputs=2
  Demux2 : Demux  Outputs=2
  Mux : Mux  Inputs=2
  Product : Product  SaturateOnIntegerOverflow=on  InputSameDT=on  OutDataTypeStr=Inherit: Same as first input
  Product1 : Product  SaturateOnIntegerOverflow=on  OutDataTypeStr=Inherit: Same as first input
  Selector : Selector  NumberOfDimensions=2  InputPortWidth=3  IndexOptions=Index vector (port),Index vector (port)  Indices=1,1
  Selector1 : Selector  NumberOfDimensions=2  InputPortWidth=3  IndexOptions=Index vector (port),Index vector (port)  Indices=1,1
  Sum : Sum  Inputs=|++  SaturateOnIntegerOverflow=on
  Sum1 : Sum  Inputs=|+-  SaturateOnIntegerOverflow=on
  m,n : Subsystem
  n,m-1 : Subsystem
  temp1 : Outport
  temp2 : Outport  Port=2
  wires:
  Product/1 -> Demux1/1
  tc/1 -> Selector/1, Selector1/1
  Selector/1 -> Product/2
  m,n/1(row) -> Selector/2
  m,n/2(col) -> Selector/3
  n,m/1 -> m,n/1(n,m), n,m-1/1(n,m)
  cp/1 -> Mux/1
  sp/1 -> Mux/2
  Mux/1 -> Product/1, Product1/1
  n,m-1/1(row) -> Selector1/2
  n,m-1/2(col) -> Selector1/3
  Selector1/1 -> Product1/2
  Product1/1 -> Demux2/1
  Sum/1 -> temp1/1
  Demux1/1 -> Sum/1
  Demux2/2 -> Sum/2
  Demux1/2 -> Sum1/1
  Sum1/1 -> temp2/1
  Demux2/1 -> Sum1/2

== system UKF_10hz/Orbital Enviroment/Orbital Model/Subsystem/World Magnetic Model 2010/geomag/Compute magnetic vector in spherical coordinates/For Iterator Subsystem/Compute unnormalized associated  legendre polynomials and  derivatives via recursion relations/If Action Subsystem/calculate  index ==
  n,m : Inport
  Constant : Constant  OutDataTypeStr=Inherit: Inherit via back propagation
  Demux8 : Demux  Outputs=2
  Gain : Gain  Gain=maxdef+1  SaturateOnIntegerOverflow=on  OutDataTypeStr=Inherit: Same as input  ParamDataTypeStr=Inherit: Same as input
  Sum1 : Sum  Inputs=|++  SaturateOnIntegerOverflow=on
  Sum2 : Sum  Inputs=|+-  SaturateOnIntegerOverflow=on
  e : Outport
  wires:
  Gain/1 -> Sum1/2
  Demux8/1 -> Sum1/1
  Demux8/2 -> Sum2/1
  n,m/1 -> Demux8/1
  Sum1/1 -> e/1
  Sum2/1 -> Gain/1
  Constant/1 -> Sum2/2

== system UKF_10hz/Orbital Enviroment/Orbital Model/Subsystem/World Magnetic Model 2010/geomag/Compute magnetic vector in spherical coordinates/For Iterator Subsystem/Compute unnormalized associated  legendre polynomials and  derivatives via recursion relations/If Action Subsystem/calculate  row and column ==
  n,m : Inport
  Demux8 : Demux  Outputs=2
  m : Outport
  n : Outport  Port=2
  wires:
  n,m/1 -> Demux8/1
  Demux8/2 -> m/1
  Demux8/1 -> n/1

== system UKF_10hz/Orbital Enviroment/Orbital Model/Subsystem/World Magnetic Model 2010/geomag/Compute magnetic vector in spherical coordinates/For Iterator Subsystem/Compute unnormalized associated  legendre polynomials and  derivatives via recursion relations/If Action Subsystem1/calculate  index ==
  n,m : Inport
  Demux8 : Demux  Outputs=2
  Gain : Gain  Gain=maxdef+1  SaturateOnIntegerOverflow=on  OutDataTypeStr=Inherit: Same as input  ParamDataTypeStr=Inherit: Same as input
  Sum1 : Sum  Inputs=|++  SaturateOnIntegerOverflow=on
  e : Outport
  wires:
  Gain/1 -> Sum1/2
  Demux8/1 -> Sum1/1
  Demux8/2 -> Gain/1
  n,m/1 -> Demux8/1
  Sum1/1 -> e/1

== system UKF_10hz/Orbital Enviroment/Orbital Model/Subsystem/World Magnetic Model 2010/geomag/Compute magnetic vector in spherical coordinates/For Iterator Subsystem/Compute unnormalized associated  legendre polynomials and  derivatives via recursion relations/If Action Subsystem1/calculate  row and column ==
  n,m : Inport
  Constant : Constant  OutDataTypeStr=Inherit: Inherit via back propagation
  Demux8 : Demux  Outputs=2
  Sum : Sum  Inputs=|++  SaturateOnIntegerOverflow=on  InputSameDT=on
  m+1 : Outport
  n : Outport  Port=2
  wires:
  Demux8/1 -> n/1
  Demux8/2 -> Sum/1
  n,m/1 -> Demux8/1
  Sum/1 -> m+1/1
  Constant/1 -> Sum/2

== system UKF_10hz/Orbital Enviroment/Orbital Model/Subsystem/World Magnetic Model 2010/geomag/Compute magnetic vector in spherical coordinates/For Iterator Subsystem/Compute unnormalized associated  legendre polynomials and  derivatives via recursion relations/If Action Subsystem2/calculate  indices ==
  n,m : Inport
  Constant1 : Constant  OutDataTypeStr=Inherit: Inherit via back propagation
  Demux8 : Demux  Outputs=2
  Gain : Gain  Gain=maxdef+1  SaturateOnIntegerOverflow=on  OutDataTypeStr=Inherit: Same as input  ParamDataTypeStr=Inherit: Same as input
  Mux : Mux  Inputs=2
  Sum1 : Sum  Inputs=|++  SaturateOnIntegerOverflow=on
  Sum2 : Sum  Inputs=|-+  SaturateOnIntegerOverflow=on
  e : Outport
  wires:
  Gain/1 -> Sum1/2
  Demux8/1 -> Sum2/2, Mux/2
  Demux8/2 -> Gain/1
  n,m/1 -> Demux8/1
  Sum1/1 -> e/1
  Constant1/1 -> Sum2/1
  Sum2/1 -> Mux/1
  Mux/1 -> Sum1/1

== system UKF_10hz/Orbital Enviroment/Orbital Model/Subsystem/World Magnetic Model 2010/geomag/Compute magnetic vector in spherical coordinates/For Iterator Subsystem/Compute unnormalized associated  legendre polynomials and  derivatives via recursion relations/If Action Subsystem2/calculate  row and column1 ==
  n,m : Inport
  Constant : Constant  OutDataTypeStr=Inherit: Inherit via back propagation
  Demux8 : Demux  Outputs=2
  Sum : Sum  Inputs=|++  SaturateOnIntegerOverflow=on
  m+1 : Outport
  n+1 : Outport  Port=2
  wires:
  Demux8/1 -> n+1/1
  Demux8/2 -> m+1/1
  n,m/1 -> Sum/1
  Constant/1 -> Sum/2
  Sum/1 -> Demux8/1

== system UKF_10hz/Orbital Enviroment/Orbital Model/Subsystem/World Magnetic Model 2010/geomag/Compute magnetic vector in spherical coordinates/For Iterator Subsystem/Compute unnormalized associated  legendre polynomials and  derivatives via recursion relations/If Action Subsystem2/calculate  row and column2 ==
  n,m : Inport
  Constant : Constant  OutDataTypeStr=Inherit: Inherit via back propagation
  Constant1 : Constant  OutDataTypeStr=Inherit: Inherit via back propagation
  Demux8 : Demux  Outputs=2
  Mux : Mux  Inputs=2
  Sum : Sum  Inputs=|++  SaturateOnIntegerOverflow=on  InputSameDT=on
  Sum2 : Sum  Inputs=|+-  SaturateOnIntegerOverflow=on
  m+1 : Outport
  n-1,n : Outport  Port=2
  wires:
  Mux/1 -> n-1,n/1
  Sum2/1 -> Mux/2
  Constant1/1 -> Sum2/2
  Demux8/1 -> Sum2/1, Mux/1
  Demux8/2 -> Sum/1
  n,m/1 -> Demux8/1
  Sum/1 -> m+1/1
  Constant/1 -> Sum/2

== system UKF_10hz/Orbital Enviroment/Orbital Model/Subsystem/World Magnetic Model 2010/geomag/Compute magnetic vector in spherical coordinates/For Iterator Subsystem/Compute unnormalized associated  legendre polynomials and  derivatives via recursion relations/If Action Subsystem2/m<n-2 ==
  n,m : Inport
  Constant1 : Constant  Value=2  OutDataTypeStr=Inherit: Inherit via back propagation
  Data Type Conversion : DataTypeConversion  SaturateOnIntegerOverflow=on  RndMeth=Zero
  Demux : Demux  Outputs=2
  Relational Operator : RelationalOperator
  Sum2 : Sum  Inputs=|+-  SaturateOnIntegerOverflow=on
  n-2>=m : Outport
  wires:
  Relational Operator/1 -> Data Type Conversion/1
  Constant1/1 -> Sum2/2
  n,m/1 -> Demux/1
  Data Type Conversion/1 -> n-2>=m/1
  Sum2/1 -> Relational Operator/1
  Demux/1 -> Sum2/1
  Demux/2 -> Relational Operator/2

== system UKF_10hz/Orbital Enviroment/Orbital Model/Subsystem/World Magnetic Model 2010/geomag/Compute magnetic vector in spherical coordinates/For Iterator Subsystem/Compute unnormalized associated  legendre polynomials and  derivatives via recursion relations/If Action Subsystem2/m<n-2  ==
  n,m : Inport
  Constant1 : Constant  Value=2  OutDataTypeStr=Inherit: Inherit via back propagation
  Data Type Conversion : DataTypeConversion  SaturateOnIntegerOverflow=on  RndMeth=Zero
  Demux : Demux  Outputs=2
  Relational Operator : RelationalOperator
  Sum2 : Sum  Inputs=|+-  SaturateOnIntegerOverflow=on
  n-2>=m : Outport
  wires:
  Relational Operator/1 -> Data Type Conversion/1
  Constant1/1 -> Sum2/2
  n,m/1 -> Demux/1
  Data Type Conversion/1 -> n-2>=m/1
  Sum2/1 -> Relational Operator/1
  Demux/1 -> Sum2/1
  Demux/2 -> Relational Operator/2

== system UKF_10hz/Orbital Enviroment/Orbital Model/Subsystem/World Magnetic Model 2010/geomag/Compute magnetic vector in spherical coordinates/For Iterator Subsystem/Time adjust the gauss coefficients/if (m~=0)/If Action Subsystem1 ==
  m : Inport
  n : Inport  Port=2
  dt : Inport  Port=3
  c : Inport  Port=4
  cd : Inport  Port=5
  tc_old : Inport  Port=6
  Action Port : ActionPort  PropagateVarSize=During execution  ActionType=then
  Assignment2 : Assignment  NumberOfDimensions=2  DiagnosticForDimensions=Error  IndexOptions=Index vector (port),Index vector (port)  Indices=1,1  OutputSizes=1,1
  Constant : Constant  OutDataTypeStr=Inherit: Inherit via back propagation
  Gain : Gain
  Product : Product  SaturateOnIntegerOverflow=on  OutDataTypeStr=Inherit: Same as first input
  Sum : Sum  Inputs=|++  SaturateOnIntegerOverflow=on
  Sum2 : Sum  Inputs=|++  SaturateOnIntegerOverflow=on  InputSameDT=on
  c[m][n] : Selector  NumberOfDimensions=2  InputPortWidth=3  IndexOptions=Index vector (port),Index vector (port)  Indices=1,1
  cd[m][n] : Selector  NumberOfDimensions=2  InputPortWidth=3  IndexOptions=Index vector (port),Index vector (port)  Indices=1,1
  tc[13][13] : Outport
  wires:
  Gain/1 -> tc[13][13]/1
  Sum/1 -> Assignment2/2
  Product/1 -> Sum/2
  c[m][n]/1 -> Sum/1
  cd[m][n]/1 -> Product/1
  dt/1 -> Product/2
  cd/1 -> cd[m][n]/1
  c/1 -> c[m][n]/1
  Sum2/1 -> c[m][n]/2, cd[m][n]/2, Assignment2/3
  m/1 -> c[m][n]/3, cd[m][n]/3, Assignment2/4
  Constant/1 -> Sum2/2
  n/1 -> Sum2/1
  tc_old/1 -> Assignment2/1
  Assignment2/1 -> Gain/1

== system UKF_10hz/Orbital Enviroment/Orbital Model/Subsystem/World Magnetic Model 2010/geomag/Compute magnetic vector in spherical coordinates/For Iterator Subsystem/Time adjust the gauss coefficients/if (m~=0)/If Action Subsystem2 ==
  tc_old : Inport
  Action Port : ActionPort  PropagateVarSize=During execution  ActionType=else
  tc[13][13] : Outport
  wires:
  tc_old/1 -> tc[13][13]/1

== system UKF_10hz/Orbital Enviroment/Orbital Model/Subsystem/World Magnetic Model 2010/geomag/Compute magnetic vector in spherical coordinates/For Iterator Subsystem/Accumulate terms of the  spherical harmonic expansion/Special case - North/South Geographic Pole/If Action Subsystem2/calculate  indices ==
  n : Inport
  Constant1 : Constant  OutDataTypeStr=Inherit: Inherit via back propagation
  Mux : Mux  Inputs=2
  Sum2 : Sum  Inputs=|-+  SaturateOnIntegerOverflow=on
  e : Outport
  wires:
  n/1 -> Sum2/2, Mux/2
  Constant1/1 -> Sum2/1
  Sum2/1 -> Mux/1
  Mux/1 -> e/1

== system UKF_10hz/Orbital Enviroment/Orbital Model/Subsystem/World Magnetic Model 2010/geomag/Compute magnetic vector in spherical coordinates/For Iterator Subsystem/Accumulate terms of the  spherical harmonic expansion/Special case - North/South Geographic Pole/If Action Subsystem2/calculate  row and column ==
  n,m : Inport
  Constant : Constant  OutDataTypeStr=Inherit: Inherit via back propagation
  Demux8 : Demux  Outputs=2
  Sum : Sum  Inputs=|++  SaturateOnIntegerOverflow=on
  m+1 : Outport
  n+1 : Outport  Port=2
  wires:
  Demux8/1 -> n+1/1
  Demux8/2 -> m+1/1
  n,m/1 -> Sum/1
  Constant/1 -> Sum/2
  Sum/1 -> Demux8/1

== system UKF_10hz/Orbital Enviroment/Orbital Model/Subsystem/World Magnetic Model 2010/geomag/Compute magnetic vector in spherical coordinates/For Iterator Subsystem/Accumulate terms of the  spherical harmonic expansion/calculate temp values/If Action Subsystem1/m,n ==
  n,m : Inport
  Constant : Constant
  Demux : Demux  Outputs=2
  Selector1 : Selector  InputPortWidth=2  Indices=[2 1]
  Sum : Sum  Inputs=|++  SaturateOnIntegerOverflow=on
  row : Outport
  col : Outport  Port=2
  wires:
  Sum/1 -> Selector1/1
  Constant/1 -> Sum/2
  Selector1/1 -> Demux/1
  Demux/1 -> row/1
  n,m/1 -> Sum/1
  Demux/2 -> col/1

== system UKF_10hz/Orbital Enviroment/Orbital Model/Subsystem/World Magnetic Model 2010/geomag/Compute magnetic vector in spherical coordinates/For Iterator Subsystem/Accumulate terms of the  spherical harmonic expansion/calculate temp values/If Action Subsystem1/n,m-1 ==
  n,m : Inport
  Constant : Constant
  Demux : Demux  Outputs=2
  Sum : Sum  Inputs=|++  SaturateOnIntegerOverflow=on
  row : Outport
  col : Outport  Port=2
  wires:
  n,m/1 -> Demux/1
  Constant/1 -> Sum/2
  Demux/1 -> Sum/1
  Sum/1 -> row/1
  Demux/2 -> col/1
